simulink model "IDM_Acceleration_Model_V2"  (R2025b)
settings: Solver=VariableStepAuto  StartTime=0.0  StopTime=20  RelTol=1e-3
libraries: SignalEditorBlockLib x1
settings Model: Creator=Ahmed  LastModifiedBy=Ahmed

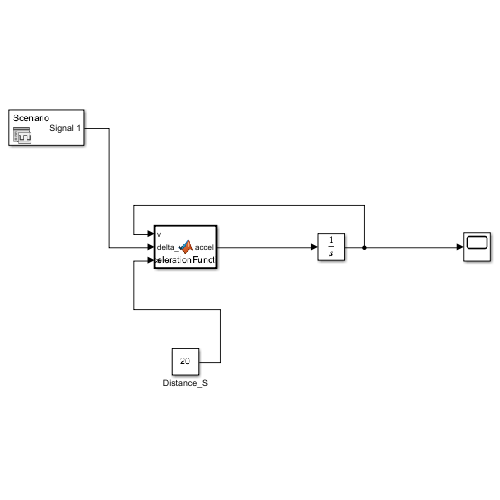
[thumbnail: Simulink's stored preview of the top-level diagram]
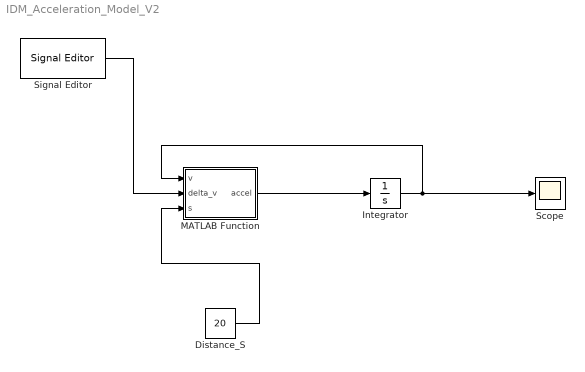
== system IDM_Acceleration_Model_V2 ==
  Distance_S : Constant  Value=20
  Integrator : Integrator
  MATLAB Function : MATLAB Function  TreatAsAtomicUnit=on
  Scope : Scope
      settings: ActiveDisplayYMinimum=-4.9914893959517883  ActiveDisplayYMaximum=17.923753429201646
  Signal Editor : SignalEditorBlockLib/Signal Editor  FileName=untitled.mat  ActiveScenario=Scenario  ActiveSignal=Signal 1  IsBus=off  OutputBusObjectStr=Bus: BusObject  SampleTime=0  ZeroCross=off  OutputAfterFinalValue=Setting to zero  Unit=inherit  PreserveSignalName=on  ApplySigPropsToAllScenarios=on  ApplySigPropsToAllSignals=off  SignalPropertySource=Dialog parameters
  wires:
  Integrator/1 -> MATLAB Function/1(v), Scope/1
  MATLAB Function/1(accel) -> Integrator/1
  Signal Editor/1 -> MATLAB Function/2(delta_v)
  Distance_S/1 -> MATLAB Function/3(s)

== matlab function IDM_Acceleration_Model_V2/MATLAB Function ==
  data: v input; accel output; delta_v input; s input
function accel = accelerationFunction(v, delta_v, s)
    % IDM Parametreleri
    a = 2;          % maksimum ivme (m/s²)
    b = -2;         % minimum yavaşlama (m/s²)
    v0 = 30;        % cruise hız (m/s)
    s0 = 2;         % jam mesafesi (m)
    T = 1.5;        % time gap (s)
    delta = 2;      % agresiflik katsayısı
    
    % Güvenli kontroller
    if s <= 0.1
        s = 0.1;    % Sıfıra bölmeyi engelle
    end
    
    if v < 0
        v = 0;      % Negatif hızı engelle
    end
    
    % s* (desired spacing) hesabı
    s_star = s0 + max(0, v*T + (v*delta_v)/(2*sqrt(abs(a*b))));
    
    % Ana IDM formülü
    accel = a * (1 - (v/v0)^delta - (s_star/s)^2);
end
